simulink model "lab1real"  (Simulink 7.9)
settings: Solver=ode45  SolverMode=SingleTasking  StartTime=0.0  StopTime=12  FixedStep=0.001  RelTol=1e-3
values from neighbouring files (symbols this model uses):
  Convert = Convert_vec(i)    [initthrottle.m]
  Convert2 = 1.95    [initthrottle.m]
  DZPOS_hat = dzpos_vec(i)    [initthrottle.m]
  fixwidth = 2    [initthrottle.m]
  h = 0.01    [initthrottle.m]
  lK = lK'    [initthrottle.m]
  lLc = 0.1    [initthrottle.m]
  lLe = place(lphie,lgame,roots(pd))    [initthrottle.m]
  Lower = Lower_vec(i)    [initthrottle.m]
  Offset = -4.7181    [initthrottle.m]
  TL_hat = tl_vec(i)    [initthrottle.m]
  TR = 100    [initthrottle.m]
  TU_hat = tu_vec(i)    [initthrottle.m]
  uK = uK'    [initthrottle.m]
  uLc = 0.1    [initthrottle.m]
  uLe = place(uphie,ugame,roots(pd))    [initthrottle.m]
undefined symbols (not defined in the file or in its folder): DiscIntNeverNeededParam, lC, lGAM, lPHI, uC, uGAM, uPHI
libraries: simulink x3, simulink_extras x1
settings Model: Creator=x98jg  LastModifiedBy=oloft  ExtModeTrigMode=oneshot  ExtModeArmWhenConnect=off  ExtModeAutoUpdateStatusClock=off
settings DataIOCC: LimitDataPoints=off
settings OptimizationCC: BooleanDataType=off
settings DebuggingCC: SaveWithParameterizedLinksMsg=none  SignalResolutionControl=TryResolveAllWithWarning  SolverPrmCheckMsg=none  MultiTaskDSMMsg=warning  MultiTaskCondExecSysMsg=none  UnconnectedInputMsg=none  UnconnectedOutputMsg=none  StrictBusMsg=None
settings HardwareCC: TargetUnknown=on
settings RTWCC: IncludeERTFirstTime=on
settings GRTTargetCC: CombineOutputUpdateFcns=off  GRTInterface=on

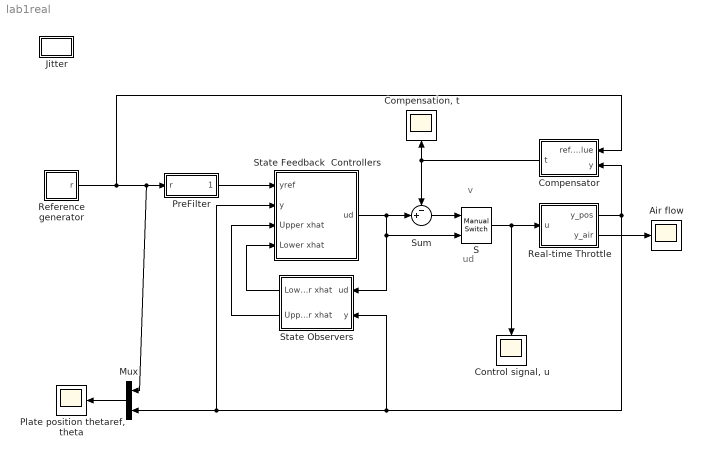
== system lab1real ==
  note: v
  note: ud
  Air flow : Scope
      settings: TimeRange=12  YMin=17.5  YMax=45
  "Compensation, t" : Scope
      settings: TimeRange=20  YMin=-1.25  YMax=1
  Compensator : Subsystem
  "Control signal, u" : Scope
      settings: TimeRange=12  YMin=0.8  YMax=2
  Jitter : Subsystem
  Mux : Mux  Inputs=2
  "Plate position thetaref, theta" : Scope
      settings: TimeRange=12  YMin=17.5  YMax=45
  PreFilter : Subsystem
  Real-time Throttle : Subsystem
  Reference generator : Subsystem
  S : simulink/Signal Routing/Manual Switch  sw=1  action=0  varsize=off
  "State Feedback  Controllers " : Subsystem
  State Observers : Subsystem
  Sum : Sum  Inputs=-+|  SaturateOnIntegerOverflow=on  InputSameDT=on  OutDataTypeStr=Inherit: Same as first input
  wires:
  State Observers/1(Lower xhat) -> "State Feedback  Controllers "/4(Lower xhat)
  State Observers/2(Upper xhat) -> "State Feedback  Controllers "/3(Upper xhat)
  Sum/1 -> S/1
  "State Feedback  Controllers "/1(ud) -> Sum/2, S/2, State Observers/1(ud)
  Real-time Throttle/1(y_pos) -> Mux/2, "State Feedback  Controllers "/2(y), State Observers/2(y), Compensator/2(y)
  Compensator/1(t) -> Sum/1, "Compensation, t"/1
  Mux/1 -> "Plate position thetaref, theta"/1
  Reference generator/1(r) -> Compensator/1(ref. value), PreFilter/1(r), Mux/1
  S/1 -> "Control signal, u"/1, Real-time Throttle/1(u)
  PreFilter/1(rfiltered) -> "State Feedback  Controllers "/1(yref)
  Real-time Throttle/2(y_air) -> Air flow/1

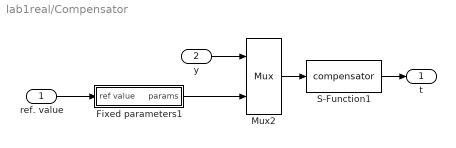
== system lab1real/Compensator ==
  ref. value : Inport
  y : Inport  Port=2
  Fixed parameters1 : Subsystem
  Mux2 : Mux  Inputs=2
  S-Function1 : S-Function  FunctionName=compensator  Parameters=h 0*fixwidth/2 -0*fixwidth/2  EnableBusSupport=off
  t : Outport
  wires:
  Fixed parameters1/1(params) -> Mux2/2
  ref. value/1 -> Fixed parameters1/1(ref value)
  y/1 -> Mux2/1
  S-Function1/1 -> t/1
  Mux2/1 -> S-Function1/1

== system lab1real/Jitter ==
  Jitter plot : Scope
      settings: TimeRange=10  YMin=5.55112e-17  YMax=1
  S-Function1 : S-Function  FunctionName=realtimer  Parameters=h  EnableBusSupport=off
  wires:
  S-Function1/1 -> Jitter plot/1

== system lab1real/PreFilter ==
  r : Inport
  Prefilter (with initial outputs=0) : simulink_extras/Additional Discrete/Discrete Transfer Fcn (with initial outputs)  N=[21.3 1 -20.3]  D=[835 -1596 763]  U0=[DZPOS_hat]  Y0=DZPOS_hat  TS=h
  rfiltered : Outport
  wires:
  Prefilter (with initial outputs=0)/1 -> rfiltered/1
  r/1 -> Prefilter (with initial outputs=0)/1

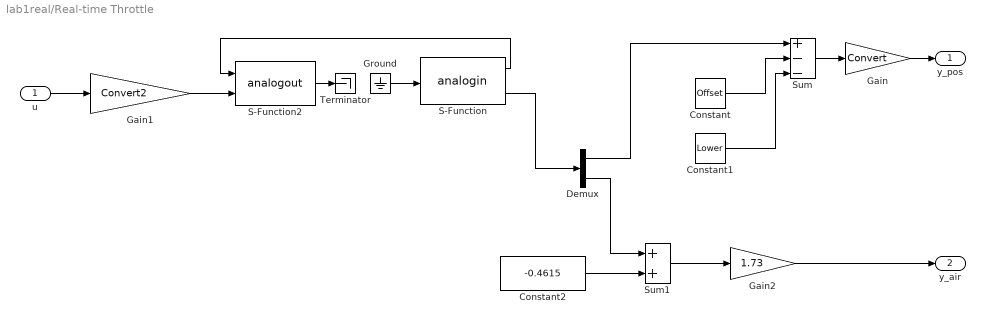
== system lab1real/Real-time Throttle ==
  u : Inport
  Constant : Constant  Value=Offset
  Constant1 : Constant  Value=Lower
  Constant2 : Constant  Value=-0.4615
  Demux : Demux  Outputs=2
  Gain : Gain  Gain=Convert  SaturateOnIntegerOverflow=on  OutDataTypeStr=Inherit: Same as input  ParamDataTypeStr=Inherit: Same as input
  Gain1 : Gain  Gain=Convert2  SaturateOnIntegerOverflow=on  OutDataTypeStr=Inherit: Same as input  ParamDataTypeStr=Inherit: Same as input
  Gain2 : Gain  Gain=1.73  SaturateOnIntegerOverflow=on  OutDataTypeStr=Inherit: Same as input  ParamDataTypeStr=Inherit: Same as input
  Ground : Ground
  S-Function : S-Function  FunctionName=analogin  Parameters=h [0 1]  EnableBusSupport=off
  S-Function2 : S-Function  FunctionName=analogout  Parameters=h [0]  EnableBusSupport=off
  Sum : Sum  Inputs=+--  SaturateOnIntegerOverflow=on  InputSameDT=on  OutDataTypeStr=Inherit: Same as first input
  Sum1 : Sum  SaturateOnIntegerOverflow=on  InputSameDT=on  OutDataTypeStr=Inherit: Same as first input
  Terminator : Terminator
  y_pos : Outport
  y_air : Outport  Port=2
  wires:
  Gain/1 -> y_pos/1
  Ground/1 -> S-Function/1
  S-Function2/1 -> Terminator/1
  S-Function/1 -> S-Function2/1
  Constant/1 -> Sum/2
  Constant1/1 -> Sum/3
  Sum/1 -> Gain/1
  u/1 -> Gain1/1
  Gain1/1 -> S-Function2/2
  S-Function/2 -> Demux/1
  Demux/1 -> Sum/1
  Demux/2 -> Sum1/1
  Constant2/1 -> Sum1/2
  Sum1/1 -> Gain2/1
  Gain2/1 -> y_air/1

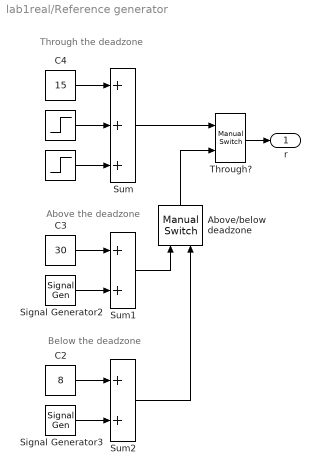
== system lab1real/Reference generator ==
  note: Through the deadzone
  note: Above the deadzone
  note: Below the deadzone
  " " : Step  Time=8  After=-6  SampleTime=0
  "  " : Step  Time=4  After=6  SampleTime=0
  Above/below deadzone : simulink/Signal Routing/Manual Switch  sw=1  action=0  varsize=off
  C2 : Constant  Value=8
  C3 : Constant  Value=30
  C4 : Constant  Value=15
  Signal Generator2 : SignalGenerator  WaveForm=square  Amplitude=-5  Frequency=0.125
  Signal Generator3 : SignalGenerator  WaveForm=square  Amplitude=5  Frequency=0.125
  Sum : Sum  Inputs=+++  SaturateOnIntegerOverflow=on  InputSameDT=on  OutDataTypeStr=Inherit: Same as first input
  Sum1 : Sum  SaturateOnIntegerOverflow=on  InputSameDT=on  OutDataTypeStr=Inherit: Same as first input
  Sum2 : Sum  SaturateOnIntegerOverflow=on  InputSameDT=on  OutDataTypeStr=Inherit: Same as first input
  Through? : simulink/Signal Routing/Manual Switch  sw=0  action=0  varsize=off
  r : Outport
  wires:
  C4/1 -> Sum/1
  " "/1 -> Sum/2
  "  "/1 -> Sum/3
  Signal Generator2/1 -> Sum1/2
  C3/1 -> Sum1/1
  C2/1 -> Sum2/1
  Signal Generator3/1 -> Sum2/2
  Through?/1 -> r/1
  Sum/1 -> Through?/1
  Sum1/1 -> Above/below deadzone/1
  Sum2/1 -> Above/below deadzone/2
  Above/below deadzone/1 -> Through?/2

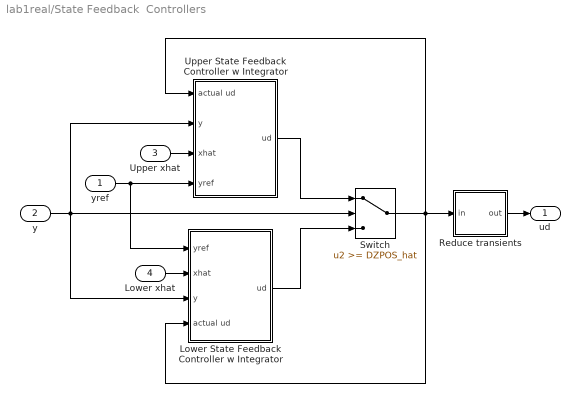
== system lab1real/State Feedback  Controllers  ==
  yref : Inport
  y : Inport  Port=2
  Upper xhat : Inport  Port=3
  Lower xhat : Inport  Port=4
  Lower State Feedback Controller w Integrator : Subsystem
  Reduce transients : Subsystem
  Switch : Switch  Threshold=DZPOS_hat  SaturateOnIntegerOverflow=on  InputSameDT=on
  Upper State Feedback Controller w Integrator : Subsystem
  ud : Outport
  wires:
  Lower State Feedback Controller w Integrator/1(ud) -> Switch/3
  Upper State Feedback Controller w Integrator/1(ud) -> Switch/1
  Lower xhat/1 -> Lower State Feedback Controller w Integrator/2(xhat)
  Switch/1 -> Lower State Feedback Controller w Integrator/4(actual ud), Reduce transients/1(in), Upper State Feedback Controller w Integrator/1(actual ud)
  Reduce transients/1(out) -> ud/1
  Upper xhat/1 -> Upper State Feedback Controller w Integrator/3(xhat)
  y/1 -> Switch/2, Upper State Feedback Controller w Integrator/2(y), Lower State Feedback Controller w Integrator/3(y)
  yref/1 -> Upper State Feedback Controller w Integrator/4(yref), Lower State Feedback Controller w Integrator/1(yref)

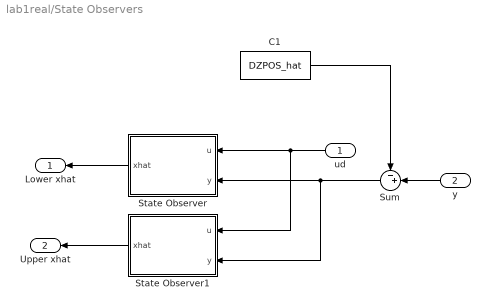
== system lab1real/State Observers ==
  ud : Inport
  y : Inport  Port=2
  C1 : Constant  Value=DZPOS_hat
  State Observer : Subsystem
  State Observer1 : Subsystem
  Sum : Sum  Inputs=-+|  SaturateOnIntegerOverflow=on  InputSameDT=on  OutDataTypeStr=Inherit: Same as first input
  Lower xhat : Outport
  Upper xhat : Outport  Port=2
  wires:
  State Observer/1(xhat) -> Lower xhat/1
  ud/1 -> State Observer/1(u), State Observer1/1(u)
  y/1 -> Sum/2
  Sum/1 -> State Observer/2(y), State Observer1/2(y)
  C1/1 -> Sum/1
  State Observer1/1(xhat) -> Upper xhat/1

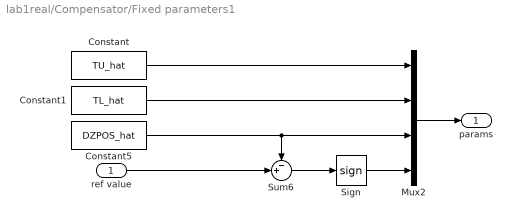
== system lab1real/Compensator/Fixed parameters1 ==
  ref value : Inport
  Constant : Constant  Value=TU_hat
  Constant1 : Constant  Value=TL_hat
  Constant5 : Constant  Value=DZPOS_hat
  Mux2 : Mux
  Sign : Signum
  Sum6 : Sum  Inputs=-+|  SaturateOnIntegerOverflow=on  InputSameDT=on  OutDataTypeStr=Inherit: Same as first input
  params : Outport
  wires:
  Sign/1 -> Mux2/4
  Constant/1 -> Mux2/1
  ref value/1 -> Sum6/2
  Constant1/1 -> Mux2/2
  Mux2/1 -> params/1
  Sum6/1 -> Sign/1
  Constant5/1 -> Mux2/3, Sum6/1

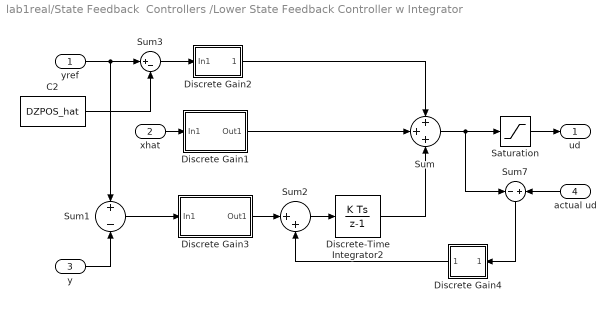
== system lab1real/State Feedback  Controllers /Lower State Feedback Controller w Integrator ==
  yref : Inport
  xhat : Inport  Port=2
  y : Inport  Port=3
  actual ud : Inport  Port=4
  C2 : Constant  Value=DZPOS_hat
  Discrete Gain1 : Subsystem  mask(Discrete Gain){h=h, K=-lLe(1:3)}
      mask prompts: h "Sample Time"; K "Gain"
      mask init:
      | s = get_param(gcb,'MaskValueString');
      | s = s(findstr(s,'|')+1:end);
      mask Display: disp(s)
  Discrete Gain2 : Subsystem  mask(Discrete Gain){h=h, K=lLc}
      mask prompts: h "Sample Time"; K "Gain"
      mask init:
      | s = get_param(gcb,'MaskValueString');
      | s = s(findstr(s,'|')+1:end);
      mask Display: disp(s)
  Discrete Gain3 : Subsystem  mask(Discrete Gain){h=h, K=-lLe(4)}
      mask prompts: h "Sample Time"; K "Gain"
      mask init:
      | s = get_param(gcb,'MaskValueString');
      | s = s(findstr(s,'|')+1:end);
      mask Display: disp(s)
  Discrete Gain4 : Subsystem  mask(Discrete Gain){h=h, K=TR}
      mask prompts: h "Sample Time"; K "Gain"
      mask init:
      | s = get_param(gcb,'MaskValueString');
      | s = s(findstr(s,'|')+1:end);
      mask Display: disp(s)
  Discrete-Time Integrator2 : DiscreteIntegrator  SampleTime=h  ICPrevOutput=DiscIntNeverNeededParam  ICPrevScaledInput=DiscIntNeverNeededParam
  Saturation : Saturate  UpperLimit=7  LowerLimit=-7
  Sum : Sum  Inputs=+++  SaturateOnIntegerOverflow=on  InputSameDT=on  OutDataTypeStr=Inherit: Same as first input
  Sum1 : Sum  Inputs=+-  SaturateOnIntegerOverflow=on  InputSameDT=on  OutDataTypeStr=Inherit: Same as first input
  Sum2 : Sum  Inputs=|++  SaturateOnIntegerOverflow=on  InputSameDT=on  OutDataTypeStr=Inherit: Same as first input
  Sum3 : Sum  Inputs=|+-  SaturateOnIntegerOverflow=on  InputSameDT=on  OutDataTypeStr=Inherit: Same as first input
  Sum7 : Sum  Inputs=-+  SaturateOnIntegerOverflow=on  InputSameDT=on  OutDataTypeStr=Inherit: Same as first input
  ud : Outport
  wires:
  Discrete Gain2/1(Out1) -> Sum/1
  xhat/1 -> Discrete Gain1/1(In1)
  Discrete Gain1/1(Out1) -> Sum/2
  Sum7/1 -> Discrete Gain4/1(In1)
  actual ud/1 -> Sum7/2
  Sum/1 -> Sum7/1, Saturation/1
  Saturation/1 -> ud/1
  Discrete-Time Integrator2/1 -> Sum/3
  Discrete Gain3/1(Out1) -> Sum2/1
  Sum2/1 -> Discrete-Time Integrator2/1
  y/1 -> Sum1/2
  Sum1/1 -> Discrete Gain3/1(In1)
  Discrete Gain4/1(Out1) -> Sum2/2
  Sum3/1 -> Discrete Gain2/1(In1)
  yref/1 -> Sum1/1, Sum3/1
  C2/1 -> Sum3/2

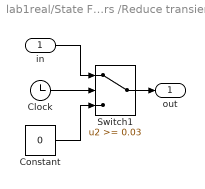
== system lab1real/State Feedback  Controllers /Reduce transients ==
  in : Inport
  Clock : Clock
  Constant : Constant  Value=0
  Switch1 : Switch  Threshold=0.03  SaturateOnIntegerOverflow=on  InputSameDT=on
  out : Outport
  wires:
  Clock/1 -> Switch1/2
  in/1 -> Switch1/1
  Switch1/1 -> out/1
  Constant/1 -> Switch1/3

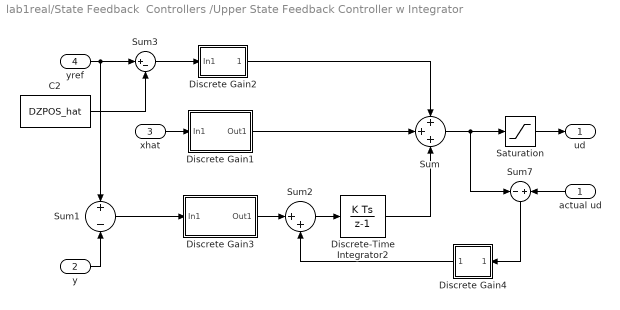
== system lab1real/State Feedback  Controllers /Upper State Feedback Controller w Integrator ==
  actual ud : Inport
  y : Inport  Port=2
  xhat : Inport  Port=3
  yref : Inport  Port=4
  C2 : Constant  Value=DZPOS_hat
  Discrete Gain1 : Subsystem  mask(Discrete Gain){h=h, K=-uLe(1:3)}
      mask prompts: h "Sample Time"; K "Gain"
      mask init:
      | s = get_param(gcb,'MaskValueString');
      | s = s(findstr(s,'|')+1:end);
      mask Display: disp(s)
  Discrete Gain2 : Subsystem  mask(Discrete Gain){h=h, K=uLc}
      mask prompts: h "Sample Time"; K "Gain"
      mask init:
      | s = get_param(gcb,'MaskValueString');
      | s = s(findstr(s,'|')+1:end);
      mask Display: disp(s)
  Discrete Gain3 : Subsystem  mask(Discrete Gain){h=h, K=-uLe(4)}
      mask prompts: h "Sample Time"; K "Gain"
      mask init:
      | s = get_param(gcb,'MaskValueString');
      | s = s(findstr(s,'|')+1:end);
      mask Display: disp(s)
  Discrete Gain4 : Subsystem  mask(Discrete Gain){h=h, K=TR}
      mask prompts: h "Sample Time"; K "Gain"
      mask init:
      | s = get_param(gcb,'MaskValueString');
      | s = s(findstr(s,'|')+1:end);
      mask Display: disp(s)
  Discrete-Time Integrator2 : DiscreteIntegrator  SampleTime=h  ICPrevOutput=DiscIntNeverNeededParam  ICPrevScaledInput=DiscIntNeverNeededParam
  Saturation : Saturate  UpperLimit=7  LowerLimit=-7
  Sum : Sum  Inputs=+++  SaturateOnIntegerOverflow=on  InputSameDT=on  OutDataTypeStr=Inherit: Same as first input
  Sum1 : Sum  Inputs=+-  SaturateOnIntegerOverflow=on  InputSameDT=on  OutDataTypeStr=Inherit: Same as first input
  Sum2 : Sum  Inputs=|++  SaturateOnIntegerOverflow=on  InputSameDT=on  OutDataTypeStr=Inherit: Same as first input
  Sum3 : Sum  Inputs=|+-  SaturateOnIntegerOverflow=on  InputSameDT=on  OutDataTypeStr=Inherit: Same as first input
  Sum7 : Sum  Inputs=-+  SaturateOnIntegerOverflow=on  InputSameDT=on  OutDataTypeStr=Inherit: Same as first input
  ud : Outport
  wires:
  xhat/1 -> Discrete Gain1/1(In1)
  Sum7/1 -> Discrete Gain4/1(In1)
  actual ud/1 -> Sum7/2
  Sum/1 -> Sum7/1, Saturation/1
  Saturation/1 -> ud/1
  Discrete Gain3/1(Out1) -> Sum2/1
  Sum2/1 -> Discrete-Time Integrator2/1
  y/1 -> Sum1/2
  Sum1/1 -> Discrete Gain3/1(In1)
  Discrete Gain4/1(Out1) -> Sum2/2
  Discrete-Time Integrator2/1 -> Sum/3
  Discrete Gain2/1(Out1) -> Sum/1
  Discrete Gain1/1(Out1) -> Sum/2
  Sum3/1 -> Discrete Gain2/1(In1)
  yref/1 -> Sum1/1, Sum3/1
  C2/1 -> Sum3/2

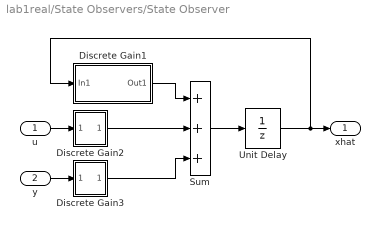
== system lab1real/State Observers/State Observer ==
  u : Inport
  y : Inport  Port=2
  Discrete Gain1 : Subsystem  mask(Discrete Gain){h=h, K=lPHI-lK*lC}
      mask prompts: h "Sample Time"; K "Gain"
      mask init:
      | s = get_param(gcb,'MaskValueString');
      | s = s(findstr(s,'|')+1:end);
      mask Display: disp(s)
  Discrete Gain2 : Subsystem  mask(Discrete Gain){h=h, K=lGAM}
      mask prompts: h "Sample Time"; K "Gain"
      mask init:
      | s = get_param(gcb,'MaskValueString');
      | s = s(findstr(s,'|')+1:end);
      mask Display: disp(s)
  Discrete Gain3 : Subsystem  mask(Discrete Gain){h=h, K=lK}
      mask prompts: h "Sample Time"; K "Gain"
      mask init:
      | s = get_param(gcb,'MaskValueString');
      | s = s(findstr(s,'|')+1:end);
      mask Display: disp(s)
  Sum : Sum  Inputs=+++  SaturateOnIntegerOverflow=on  InputSameDT=on  OutDataTypeStr=Inherit: Same as first input
  Unit Delay : UnitDelay  SampleTime=h
  xhat : Outport
  wires:
  Discrete Gain1/1(Out1) -> Sum/1
  Discrete Gain2/1(Out1) -> Sum/2
  Discrete Gain3/1(Out1) -> Sum/3
  Sum/1 -> Unit Delay/1
  Unit Delay/1 -> Discrete Gain1/1(In1), xhat/1
  u/1 -> Discrete Gain2/1(In1)
  y/1 -> Discrete Gain3/1(In1)

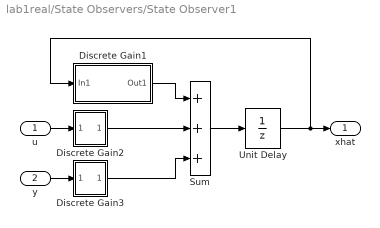
== system lab1real/State Observers/State Observer1 ==
  u : Inport
  y : Inport  Port=2
  Discrete Gain1 : Subsystem  mask(Discrete Gain){h=h, K=uPHI-uK*uC}
      mask prompts: h "Sample Time"; K "Gain"
      mask init:
      | s = get_param(gcb,'MaskValueString');
      | s = s(findstr(s,'|')+1:end);
      mask Display: disp(s)
  Discrete Gain2 : Subsystem  mask(Discrete Gain){h=h, K=uGAM}
      mask prompts: h "Sample Time"; K "Gain"
      mask init:
      | s = get_param(gcb,'MaskValueString');
      | s = s(findstr(s,'|')+1:end);
      mask Display: disp(s)
  Discrete Gain3 : Subsystem  mask(Discrete Gain){h=h, K=uK}
      mask prompts: h "Sample Time"; K "Gain"
      mask init:
      | s = get_param(gcb,'MaskValueString');
      | s = s(findstr(s,'|')+1:end);
      mask Display: disp(s)
  Sum : Sum  Inputs=+++  SaturateOnIntegerOverflow=on  InputSameDT=on  OutDataTypeStr=Inherit: Same as first input
  Unit Delay : UnitDelay  SampleTime=h
  xhat : Outport
  wires:
  Discrete Gain1/1(Out1) -> Sum/1
  Discrete Gain2/1(Out1) -> Sum/2
  Discrete Gain3/1(Out1) -> Sum/3
  Sum/1 -> Unit Delay/1
  Unit Delay/1 -> Discrete Gain1/1(In1), xhat/1
  u/1 -> Discrete Gain2/1(In1)
  y/1 -> Discrete Gain3/1(In1)

== system lab1real/State Feedback  Controllers /Lower State Feedback Controller w Integrator/Discrete Gain1 ==
  In1 : Inport
  Discrete State-Space : DiscreteStateSpace  A=0  B=zeros(1,size(K,2))  C=zeros(size(K,1),1)  D=K  SampleTime=h
  Out1 : Outport
  wires:
  Discrete State-Space/1 -> Out1/1
  In1/1 -> Discrete State-Space/1

== system lab1real/State Feedback  Controllers /Lower State Feedback Controller w Integrator/Discrete Gain2 ==
  In1 : Inport
  Discrete State-Space : DiscreteStateSpace  A=0  B=zeros(1,size(K,2))  C=zeros(size(K,1),1)  D=K  SampleTime=h
  Out1 : Outport
  wires:
  Discrete State-Space/1 -> Out1/1
  In1/1 -> Discrete State-Space/1

== system lab1real/State Feedback  Controllers /Lower State Feedback Controller w Integrator/Discrete Gain3 ==
  In1 : Inport
  Discrete State-Space : DiscreteStateSpace  A=0  B=zeros(1,size(K,2))  C=zeros(size(K,1),1)  D=K  SampleTime=h
  Out1 : Outport
  wires:
  In1/1 -> Discrete State-Space/1
  Discrete State-Space/1 -> Out1/1

== system lab1real/State Feedback  Controllers /Lower State Feedback Controller w Integrator/Discrete Gain4 ==
  In1 : Inport
  Discrete State-Space : DiscreteStateSpace  A=0  B=zeros(1,size(K,2))  C=zeros(size(K,1),1)  D=K  SampleTime=h
  Out1 : Outport
  wires:
  Discrete State-Space/1 -> Out1/1
  In1/1 -> Discrete State-Space/1

== system lab1real/State Feedback  Controllers /Upper State Feedback Controller w Integrator/Discrete Gain1 ==
  In1 : Inport
  Discrete State-Space : DiscreteStateSpace  A=0  B=zeros(1,size(K,2))  C=zeros(size(K,1),1)  D=K  SampleTime=h
  Out1 : Outport
  wires:
  Discrete State-Space/1 -> Out1/1
  In1/1 -> Discrete State-Space/1

== system lab1real/State Feedback  Controllers /Upper State Feedback Controller w Integrator/Discrete Gain2 ==
  In1 : Inport
  Discrete State-Space : DiscreteStateSpace  A=0  B=zeros(1,size(K,2))  C=zeros(size(K,1),1)  D=K  SampleTime=h
  Out1 : Outport
  wires:
  Discrete State-Space/1 -> Out1/1
  In1/1 -> Discrete State-Space/1

== system lab1real/State Feedback  Controllers /Upper State Feedback Controller w Integrator/Discrete Gain3 ==
  In1 : Inport
  Discrete State-Space : DiscreteStateSpace  A=0  B=zeros(1,size(K,2))  C=zeros(size(K,1),1)  D=K  SampleTime=h
  Out1 : Outport
  wires:
  In1/1 -> Discrete State-Space/1
  Discrete State-Space/1 -> Out1/1

== system lab1real/State Feedback  Controllers /Upper State Feedback Controller w Integrator/Discrete Gain4 ==
  In1 : Inport
  Discrete State-Space : DiscreteStateSpace  A=0  B=zeros(1,size(K,2))  C=zeros(size(K,1),1)  D=K  SampleTime=h
  Out1 : Outport
  wires:
  Discrete State-Space/1 -> Out1/1
  In1/1 -> Discrete State-Space/1

== system lab1real/State Observers/State Observer/Discrete Gain1 ==
  In1 : Inport
  Discrete State-Space : DiscreteStateSpace  A=0  B=zeros(1,size(K,2))  C=zeros(size(K,1),1)  D=K  SampleTime=h
  Out1 : Outport
  wires:
  Discrete State-Space/1 -> Out1/1
  In1/1 -> Discrete State-Space/1

== system lab1real/State Observers/State Observer/Discrete Gain2 ==
  In1 : Inport
  Discrete State-Space : DiscreteStateSpace  A=0  B=zeros(1,size(K,2))  C=zeros(size(K,1),1)  D=K  SampleTime=h
  Out1 : Outport
  wires:
  In1/1 -> Discrete State-Space/1
  Discrete State-Space/1 -> Out1/1

== system lab1real/State Observers/State Observer/Discrete Gain3 ==
  In1 : Inport
  Discrete State-Space : DiscreteStateSpace  A=0  B=zeros(1,size(K,2))  C=zeros(size(K,1),1)  D=K  SampleTime=h
  Out1 : Outport
  wires:
  Discrete State-Space/1 -> Out1/1
  In1/1 -> Discrete State-Space/1

== system lab1real/State Observers/State Observer1/Discrete Gain1 ==
  In1 : Inport
  Discrete State-Space : DiscreteStateSpace  A=0  B=zeros(1,size(K,2))  C=zeros(size(K,1),1)  D=K  SampleTime=h
  Out1 : Outport
  wires:
  Discrete State-Space/1 -> Out1/1
  In1/1 -> Discrete State-Space/1

== system lab1real/State Observers/State Observer1/Discrete Gain2 ==
  In1 : Inport
  Discrete State-Space : DiscreteStateSpace  A=0  B=zeros(1,size(K,2))  C=zeros(size(K,1),1)  D=K  SampleTime=h
  Out1 : Outport
  wires:
  In1/1 -> Discrete State-Space/1
  Discrete State-Space/1 -> Out1/1

== system lab1real/State Observers/State Observer1/Discrete Gain3 ==
  In1 : Inport
  Discrete State-Space : DiscreteStateSpace  A=0  B=zeros(1,size(K,2))  C=zeros(size(K,1),1)  D=K  SampleTime=h
  Out1 : Outport
  wires:
  Discrete State-Space/1 -> Out1/1
  In1/1 -> Discrete State-Space/1
